simulink model "four_bots_CNN_DSM_compare"  (R2021a)
settings: Solver=ode5  StartTime=0.0  StopTime=30.0  FixedStep=0.001  RelTol=1e-3
(part 1 of 2)
settings Model: Creator=a1752760  LastModifiedBy=a1752760
settings SolverCC: AlgebraicLoopSolver=TrustRegion
settings DataIOCC: ReturnWorkspaceOutputs=off
settings DebuggingCC: SFMachineParentedDataDiag=warning  ArithmeticOperatorsInVariantConditions=warning
settings SFSimCC: CustomCodeUndefinedFunction=UseInterfaceOnly

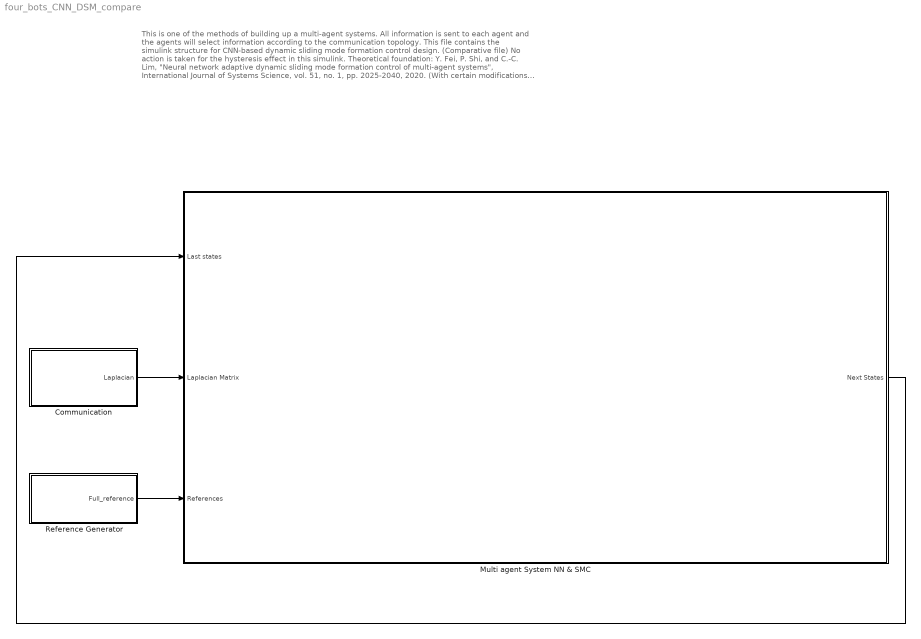
== system four_bots_CNN_DSM_compare ==
  note: This is one of the methods of building up a multi-agent systems. All information is sent to each agent and the agents will select information according to the communication topology.
      | This file contains the simulink structure for CNN-based dynamic sliding mode formation control design. (Comparative file)
      | No action is taken for the hysteresis effect in this simulink.
      | Theoretical foundation: Y. Fei, P. Shi, and C.-C. Lim, "Neural network adaptive dynamic sliding mode formation control of multi-agent systems", International Journal of Systems Science, vol. 51, no. 1, pp. 2025-2040, 2020. (With certain modifications in this simulink)
      | Note that some corrections have been made to the model (the system modelling and the formation reference part).
      | Copyright: Yang Fei @ The University of Adelaide 2021
  Communication : Subsystem
  Multi agent System NN & SMC : Subsystem
  Reference Generator : Subsystem
  wires:
  Communication/1(Laplacian) -> Multi agent System NN & SMC/2(Laplacian Matrix)
  Reference Generator/1(Full_reference) -> Multi agent System NN & SMC/3("References ")
  Multi agent System NN & SMC/1(Next States) -> Multi agent System NN & SMC/1(Last states)

== system four_bots_CNN_DSM_compare/Communication ==
  Add : Sum
  Communication Topology : Constant  Value=[2,-1,0,-1;-1,2,-1,0;0,-1,2,-1;-1,0,-1,2]  VectorParams1D=off
  Constant : Constant  Value=2  VectorParams1D=off
  Product : Product
  Reference Feeding : Constant  Value=[1,0,0,0;0,1,0,0;0,0,1,0;0,0,0,1]  VectorParams1D=off
  Laplacian : Outport  VectorParamsAs1DForOutWhenUnconnected=off
  wires:
  Constant/1 -> Product/2
  Reference Feeding/1 -> Product/1
  Communication Topology/1 -> Add/1
  Product/1 -> Add/2
  Add/1 -> Laplacian/1

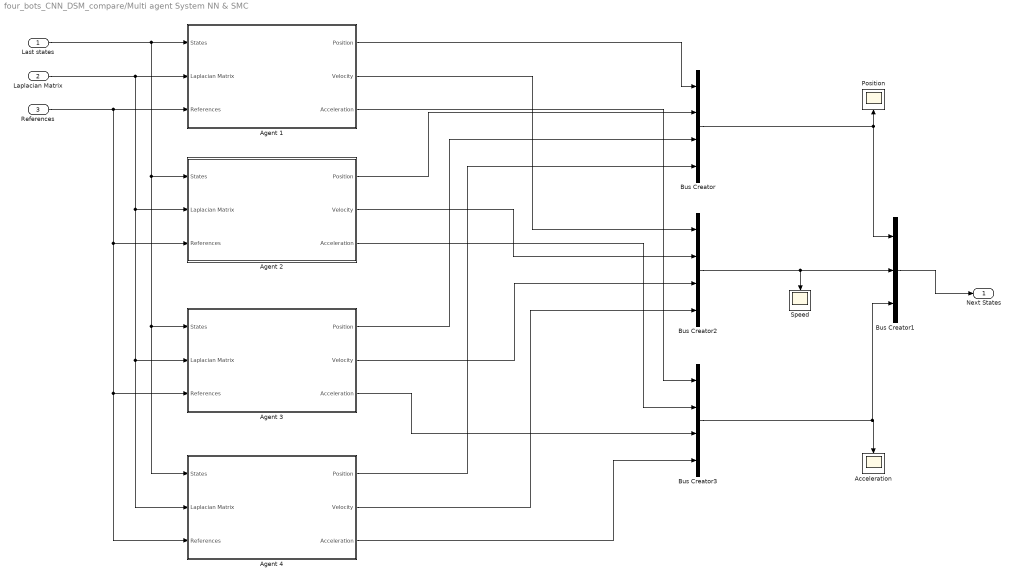
== system four_bots_CNN_DSM_compare/Multi agent System NN & SMC ==
  Last states : Inport
  Laplacian Matrix : Inport  Port=2
  "References " : Inport  Port=3
  Acceleration : Scope
  "Agent 1 " : Subsystem
  Agent 2 : Subsystem
  Agent 3 : Subsystem
  Agent 4 : Subsystem
  Bus Creator : BusCreator  Inputs=4
  Bus Creator1 : BusCreator  Inputs=3
  Bus Creator2 : BusCreator  Inputs=4
  Bus Creator3 : BusCreator  Inputs=4
  Position : Scope
  Speed : Scope
  Next States : Outport  VectorParamsAs1DForOutWhenUnconnected=off
  wires:
  Bus Creator1/1 -> Next States/1
  Last states/1 -> Agent 2/1(States), Agent 4/1(States), Agent 3/1(States), "Agent 1 "/1(States)
  Laplacian Matrix/1 -> Agent 2/2(Laplacian Matrix), Agent 4/2(Laplacian Matrix), Agent 3/2(Laplacian Matrix), "Agent 1 "/2(Laplacian Matrix)
  "References "/1 -> Agent 2/3("References "), Agent 4/3("References "), Agent 3/3("References "), "Agent 1 "/3("References ")
  "Agent 1 "/1(Position) -> Bus Creator/1
  Agent 2/1(Position) -> Bus Creator/2
  Agent 3/1(Position) -> Bus Creator/3
  Agent 4/1(Position) -> Bus Creator/4
  "Agent 1 "/2(Velocity) -> Bus Creator2/1
  Agent 2/2(Velocity) -> Bus Creator2/2
  Agent 3/2(Velocity) -> Bus Creator2/3
  Agent 4/2(Velocity) -> Bus Creator2/4
  "Agent 1 "/3(Acceleration) -> Bus Creator3/1
  Agent 2/3(Acceleration) -> Bus Creator3/2
  Agent 3/3(Acceleration) -> Bus Creator3/3
  Agent 4/3(Acceleration) -> Bus Creator3/4
  Bus Creator/1 -> Bus Creator1/1, Position/1
  Bus Creator2/1 -> Speed/1, Bus Creator1/2
  Bus Creator3/1 -> Bus Creator1/3, Acceleration/1

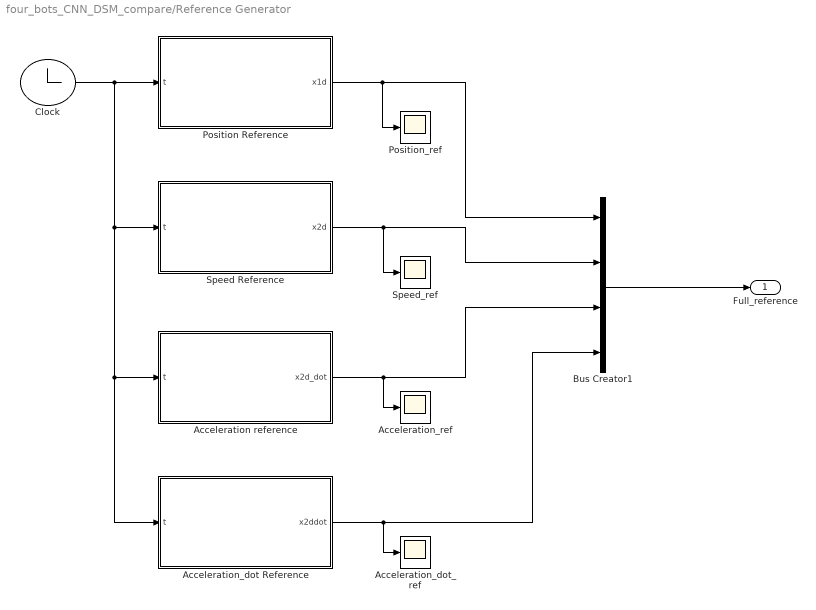
== system four_bots_CNN_DSM_compare/Reference Generator ==
  Acceleration reference : MATLAB Function  TreatAsAtomicUnit=on
  Acceleration_dot Reference : MATLAB Function  TreatAsAtomicUnit=on
  Acceleration_dot_ref : Scope
  Acceleration_ref : Scope
  Bus Creator1 : BusCreator  Inputs=4
  Clock : Clock
  Position Reference : MATLAB Function  TreatAsAtomicUnit=on
  Position_ref : Scope
  Speed Reference : MATLAB Function  TreatAsAtomicUnit=on
  Speed_ref : Scope
  Full_reference : Outport  VectorParamsAs1DForOutWhenUnconnected=off
  wires:
  Clock/1 -> Acceleration_dot Reference/1(t), Acceleration reference/1(t), Speed Reference/1(t), Position Reference/1(t)
  Position Reference/1(x1d) -> Position_ref/1, Bus Creator1/1
  Speed Reference/1(x2d) -> Speed_ref/1, Bus Creator1/2
  Acceleration reference/1(x2d_dot) -> Acceleration_ref/1, Bus Creator1/3
  Acceleration_dot Reference/1(x2ddot) -> Acceleration_dot_ref/1, Bus Creator1/4
  Bus Creator1/1 -> Full_reference/1

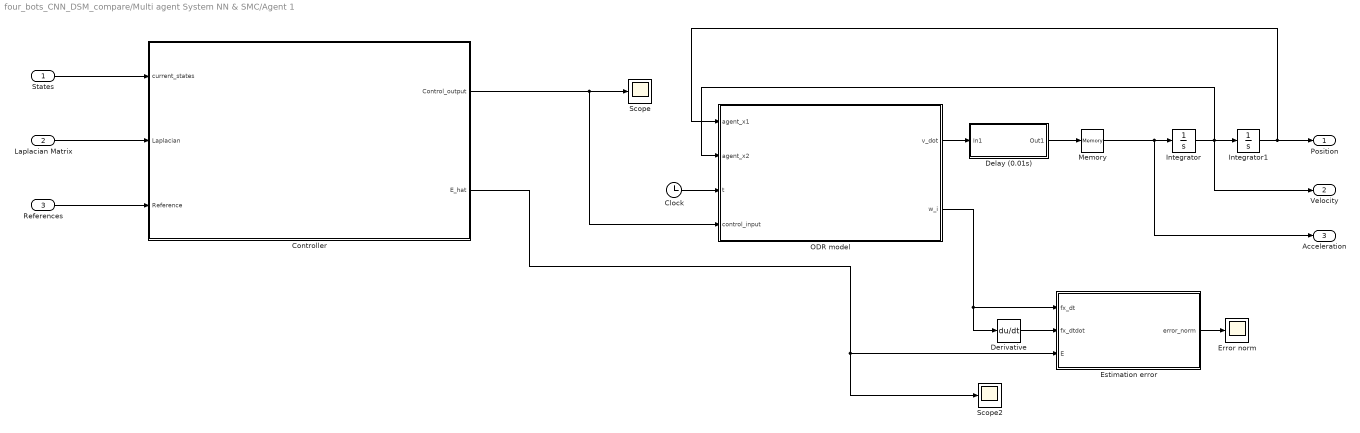
== system four_bots_CNN_DSM_compare/Multi agent System NN & SMC/Agent 1  ==
  States : Inport
  Laplacian Matrix : Inport  Port=2
  "References " : Inport  Port=3
  Clock : Clock
  "Controller " : Subsystem
  Delay (0.01s) : Subsystem
  Derivative : Derivative
  Error norm : Scope
  Estimation error : MATLAB Function  TreatAsAtomicUnit=on
  Integrator : Integrator  InitialCondition=[0;0;0]  ContinuousStateAttributes='speed'
  Integrator1 : Integrator  Tag=Position_x1  InitialCondition=[2;3;0]  ContinuousStateAttributes='position'
  Memory : Memory  InitialCondition=[0;0;0]  LinearizeMemory=on
  ODR model : MATLAB Function  TreatAsAtomicUnit=on
  Scope : Scope
  Scope2 : Scope
  Position : Outport  VectorParamsAs1DForOutWhenUnconnected=off
  Velocity : Outport  Port=2  VectorParamsAs1DForOutWhenUnconnected=off
  Acceleration : Outport  Port=3  VectorParamsAs1DForOutWhenUnconnected=off
  wires:
  ODR model/2(w_i) -> Estimation error/1(fx_dt), Derivative/1
  Integrator/1 -> ODR model/2(agent_x2), Velocity/1, Integrator1/1
  Integrator1/1 -> ODR model/1(agent_x1), Position/1
  ODR model/1(v_dot) -> Delay (0.01s)/1(In1)
  Delay (0.01s)/1(Out1) -> Memory/1
  States/1 -> "Controller "/1(current_states)
  Laplacian Matrix/1 -> "Controller "/2(Laplacian)
  "References "/1 -> "Controller "/3(Reference)
  "Controller "/1(Control_output) -> ODR model/4(control_input), Scope/1
  Clock/1 -> ODR model/3(t)
  Derivative/1 -> Estimation error/2(fx_dtdot)
  "Controller "/2(E_hat) -> Scope2/1, Estimation error/3(E)
  Estimation error/1(error_norm) -> Error norm/1
  Memory/1 -> Acceleration/1, Integrator/1

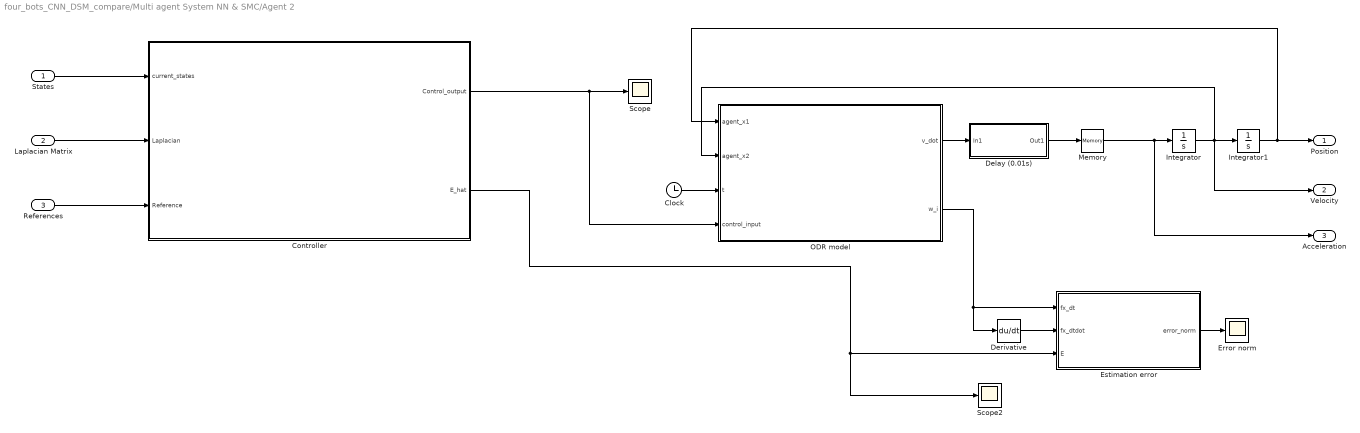
== system four_bots_CNN_DSM_compare/Multi agent System NN & SMC/Agent 2 ==
  States : Inport
  Laplacian Matrix : Inport  Port=2
  "References " : Inport  Port=3
  Clock : Clock
  "Controller " : Subsystem
  Delay (0.01s) : Subsystem
  Derivative : Derivative
  Error norm : Scope
  Estimation error : MATLAB Function  TreatAsAtomicUnit=on
  Integrator : Integrator  InitialCondition=[0;0;0]  ContinuousStateAttributes='speed'
  Integrator1 : Integrator  Tag=Position_x1  InitialCondition=[-0.5;2;pi/4]  ContinuousStateAttributes='position'
  Memory : Memory  InitialCondition=[0;0;0]  LinearizeMemory=on
  ODR model : MATLAB Function  TreatAsAtomicUnit=on
  Scope : Scope
  Scope2 : Scope
  Position : Outport  VectorParamsAs1DForOutWhenUnconnected=off
  Velocity : Outport  Port=2  VectorParamsAs1DForOutWhenUnconnected=off
  Acceleration : Outport  Port=3  VectorParamsAs1DForOutWhenUnconnected=off
  wires:
  ODR model/2(w_i) -> Estimation error/1(fx_dt), Derivative/1
  Integrator/1 -> ODR model/2(agent_x2), Velocity/1, Integrator1/1
  Integrator1/1 -> ODR model/1(agent_x1), Position/1
  ODR model/1(v_dot) -> Delay (0.01s)/1(In1)
  Delay (0.01s)/1(Out1) -> Memory/1
  States/1 -> "Controller "/1(current_states)
  Laplacian Matrix/1 -> "Controller "/2(Laplacian)
  "References "/1 -> "Controller "/3(Reference)
  "Controller "/1(Control_output) -> ODR model/4(control_input), Scope/1
  Clock/1 -> ODR model/3(t)
  Derivative/1 -> Estimation error/2(fx_dtdot)
  "Controller "/2(E_hat) -> Scope2/1, Estimation error/3(E)
  Estimation error/1(error_norm) -> Error norm/1
  Memory/1 -> Acceleration/1, Integrator/1

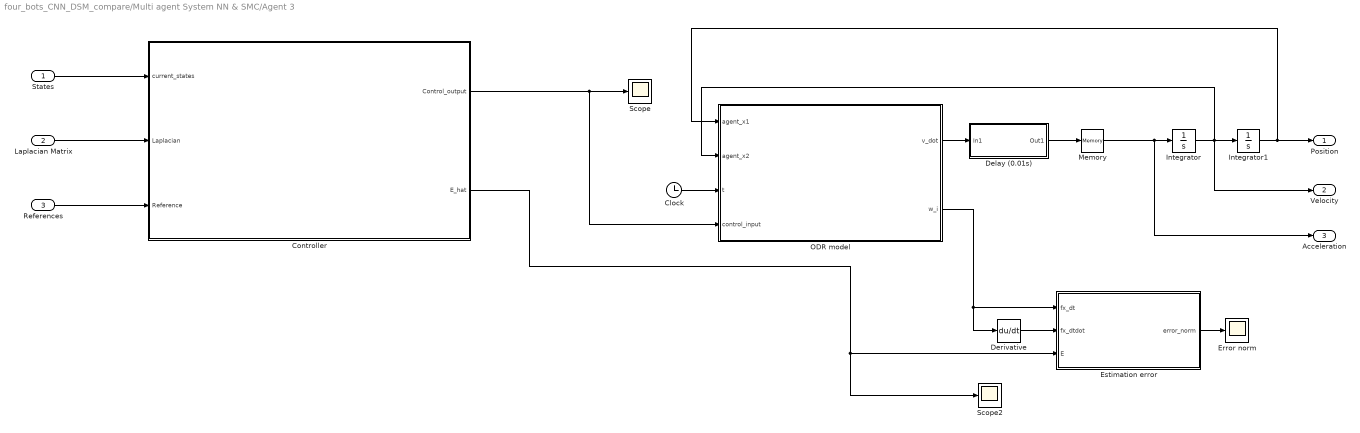
== system four_bots_CNN_DSM_compare/Multi agent System NN & SMC/Agent 3 ==
  States : Inport
  Laplacian Matrix : Inport  Port=2
  "References " : Inport  Port=3
  Clock : Clock
  "Controller " : Subsystem
  Delay (0.01s) : Subsystem
  Derivative : Derivative
  Error norm : Scope
  Estimation error : MATLAB Function  TreatAsAtomicUnit=on
  Integrator : Integrator  InitialCondition=[0;0;0]  ContinuousStateAttributes='speed'
  Integrator1 : Integrator  Tag=Position_x1  InitialCondition=[0.5;0;2*pi/3]  ContinuousStateAttributes='position'
  Memory : Memory  InitialCondition=[0;0;0]  LinearizeMemory=on
  ODR model : MATLAB Function  TreatAsAtomicUnit=on
  Scope : Scope
  Scope2 : Scope
  Position : Outport  VectorParamsAs1DForOutWhenUnconnected=off
  Velocity : Outport  Port=2  VectorParamsAs1DForOutWhenUnconnected=off
  Acceleration : Outport  Port=3  VectorParamsAs1DForOutWhenUnconnected=off
  wires:
  ODR model/2(w_i) -> Estimation error/1(fx_dt), Derivative/1
  Integrator/1 -> ODR model/2(agent_x2), Velocity/1, Integrator1/1
  Integrator1/1 -> ODR model/1(agent_x1), Position/1
  ODR model/1(v_dot) -> Delay (0.01s)/1(In1)
  Delay (0.01s)/1(Out1) -> Memory/1
  States/1 -> "Controller "/1(current_states)
  Laplacian Matrix/1 -> "Controller "/2(Laplacian)
  "References "/1 -> "Controller "/3(Reference)
  "Controller "/1(Control_output) -> ODR model/4(control_input), Scope/1
  Clock/1 -> ODR model/3(t)
  Derivative/1 -> Estimation error/2(fx_dtdot)
  "Controller "/2(E_hat) -> Scope2/1, Estimation error/3(E)
  Estimation error/1(error_norm) -> Error norm/1
  Memory/1 -> Acceleration/1, Integrator/1

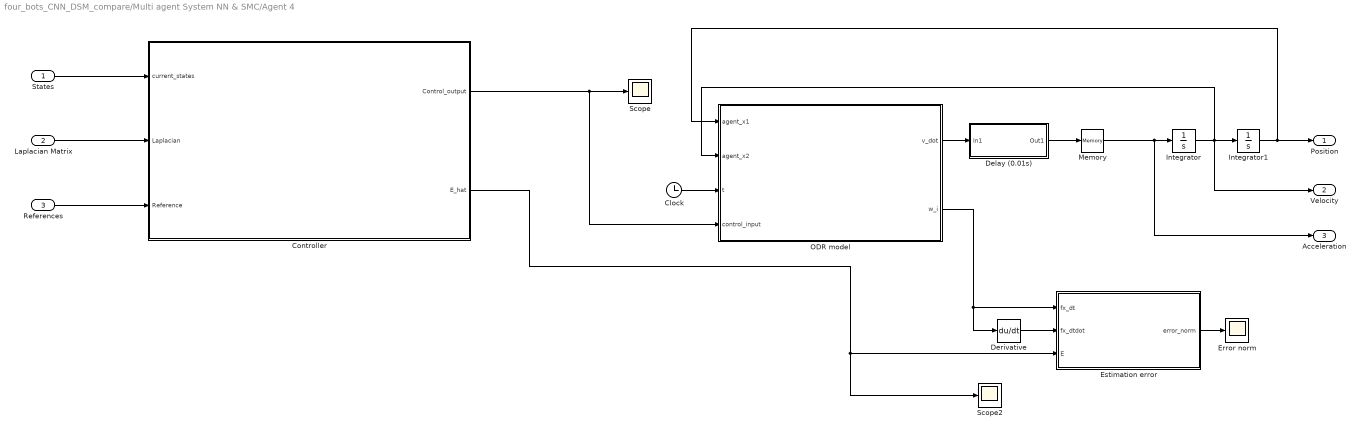
== system four_bots_CNN_DSM_compare/Multi agent System NN & SMC/Agent 4 ==
  States : Inport
  Laplacian Matrix : Inport  Port=2
  "References " : Inport  Port=3
  Clock : Clock
  "Controller " : Subsystem
  Delay (0.01s) : Subsystem
  Derivative : Derivative
  Error norm : Scope
  Estimation error : MATLAB Function  TreatAsAtomicUnit=on
  Integrator : Integrator  InitialCondition=[0;0;0]  ContinuousStateAttributes='speed'
  Integrator1 : Integrator  Tag=Position_x1  InitialCondition=[1.5;1;5*pi/4]  ContinuousStateAttributes='position'
  Memory : Memory  InitialCondition=[0;0;0]  LinearizeMemory=on
  ODR model : MATLAB Function  TreatAsAtomicUnit=on
  Scope : Scope
  Scope2 : Scope
  Position : Outport  VectorParamsAs1DForOutWhenUnconnected=off
  Velocity : Outport  Port=2  VectorParamsAs1DForOutWhenUnconnected=off
  Acceleration : Outport  Port=3  VectorParamsAs1DForOutWhenUnconnected=off
  wires:
  ODR model/2(w_i) -> Estimation error/1(fx_dt), Derivative/1
  Integrator/1 -> ODR model/2(agent_x2), Velocity/1, Integrator1/1
  Integrator1/1 -> ODR model/1(agent_x1), Position/1
  ODR model/1(v_dot) -> Delay (0.01s)/1(In1)
  Delay (0.01s)/1(Out1) -> Memory/1
  States/1 -> "Controller "/1(current_states)
  Laplacian Matrix/1 -> "Controller "/2(Laplacian)
  "References "/1 -> "Controller "/3(Reference)
  "Controller "/1(Control_output) -> ODR model/4(control_input), Scope/1
  Clock/1 -> ODR model/3(t)
  Derivative/1 -> Estimation error/2(fx_dtdot)
  "Controller "/2(E_hat) -> Scope2/1, Estimation error/3(E)
  Estimation error/1(error_norm) -> Error norm/1
  Memory/1 -> Acceleration/1, Integrator/1

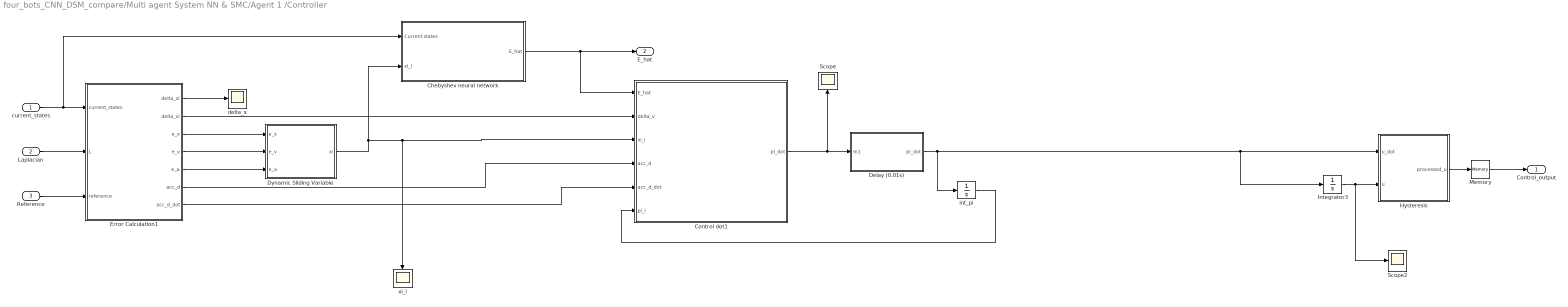
== system four_bots_CNN_DSM_compare/Multi agent System NN & SMC/Agent 1 /Controller  ==
  current_states : Inport
  Laplacian : Inport  Port=2
  Reference : Inport  Port=3
  Chebyshev neural network : Subsystem
  Control dot1 : MATLAB Function  TreatAsAtomicUnit=on
  Delay (0.01s) : Subsystem
  Dynamic Sliding Variable : MATLAB Function  TreatAsAtomicUnit=on
  Error Calculation1 : MATLAB Function  TreatAsAtomicUnit=on
  Hysteresis : Subsystem
  Integrator3 : Integrator  InitialCondition=[0;0;0]  UpperSaturationLimit=200  LowerSaturationLimit=-200  ContinuousStateAttributes='Control_output'
  Memory : Memory  InitialCondition=[0;0;0]  LinearizeMemory=on
  Scope : Scope
  Scope2 : Scope
  delta_x : Scope
  int_pi : Integrator  InitialCondition=[0;0;0]  UpperSaturationLimit=200  LowerSaturationLimit=-200  ContinuousStateAttributes='Control_output'
  xi_i : Scope
  Control_output : Outport
  E_hat : Outport  Port=2
  wires:
  Control dot1/1(pi_dot) -> Scope/1, Delay (0.01s)/1(In1)
  Hysteresis/1(processed_u) -> Memory/1
  Delay (0.01s)/1(pi_dot) -> Integrator3/1, Hysteresis/1(u_dot), int_pi/1
  Memory/1 -> Control_output/1
  Error Calculation1/4(e_v) -> Dynamic Sliding Variable/2(e_v)
  Laplacian/1 -> Error Calculation1/2(L)
  Error Calculation1/7(acc_d_dot) -> Control dot1/5(acc_d_dot)
  Error Calculation1/6(acc_d) -> Control dot1/4(acc_d)
  Reference/1 -> Error Calculation1/3(reference)
  Error Calculation1/5(e_a) -> Dynamic Sliding Variable/3(e_a)
  Error Calculation1/3(e_x) -> Dynamic Sliding Variable/1(e_x)
  Error Calculation1/2(delta_vi) -> Control dot1/2(delta_v)
  current_states/1 -> Chebyshev neural network/1(Current states), Error Calculation1/1(current_states)
  Error Calculation1/1(delta_xi) -> delta_x/1
  Dynamic Sliding Variable/1(xi) -> Control dot1/3(xi_i), xi_i/1, Chebyshev neural network/2(xi_i)
  Chebyshev neural network/1(E_hat) -> E_hat/1, Control dot1/1(E_hat)
  int_pi/1 -> Control dot1/6(pi_i)
  Integrator3/1 -> Scope2/1, Hysteresis/2(u)

== system four_bots_CNN_DSM_compare/Multi agent System NN & SMC/Agent 1 /Delay (0.01s) ==
  In1 : Inport
  Clock : Clock
  Constant : Constant  Value=[0;0;0]
  Scope3 : Scope
  Switch : Switch  Criteria=u2 > Threshold  Threshold=0.01
  Out1 : Outport  VectorParamsAs1DForOutWhenUnconnected=off
  wires:
  Constant/1 -> Switch/3
  In1/1 -> Switch/1
  Switch/1 -> Out1/1, Scope3/1
  Clock/1 -> Switch/2

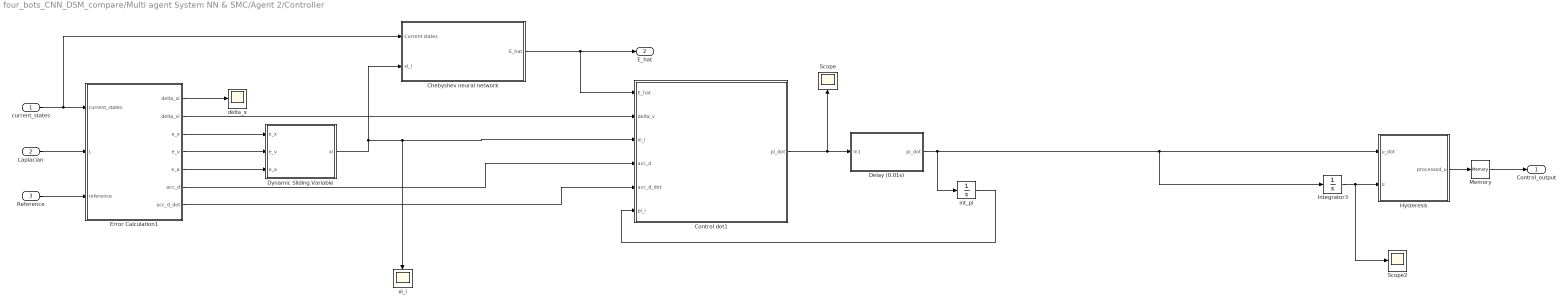
== system four_bots_CNN_DSM_compare/Multi agent System NN & SMC/Agent 2/Controller  ==
  current_states : Inport
  Laplacian : Inport  Port=2
  Reference : Inport  Port=3
  Chebyshev neural network : Subsystem
  Control dot1 : MATLAB Function  TreatAsAtomicUnit=on
  Delay (0.01s) : Subsystem
  Dynamic Sliding Variable : MATLAB Function  TreatAsAtomicUnit=on
  Error Calculation1 : MATLAB Function  TreatAsAtomicUnit=on
  Hysteresis : Subsystem
  Integrator3 : Integrator  InitialCondition=[0;0;0]  UpperSaturationLimit=200  LowerSaturationLimit=-200  ContinuousStateAttributes='Control_output'
  Memory : Memory  InitialCondition=[0;0;0]  LinearizeMemory=on
  Scope : Scope
  Scope2 : Scope
  delta_x : Scope
  int_pi : Integrator  InitialCondition=[0;0;0]  UpperSaturationLimit=200  LowerSaturationLimit=-200  ContinuousStateAttributes='Control_output'
  xi_i : Scope
  Control_output : Outport
  E_hat : Outport  Port=2
  wires:
  Control dot1/1(pi_dot) -> Scope/1, Delay (0.01s)/1(In1)
  Hysteresis/1(processed_u) -> Memory/1
  Delay (0.01s)/1(pi_dot) -> Integrator3/1, Hysteresis/1(u_dot), int_pi/1
  Memory/1 -> Control_output/1
  Error Calculation1/4(e_v) -> Dynamic Sliding Variable/2(e_v)
  Laplacian/1 -> Error Calculation1/2(L)
  Error Calculation1/7(acc_d_dot) -> Control dot1/5(acc_d_dot)
  Error Calculation1/6(acc_d) -> Control dot1/4(acc_d)
  Reference/1 -> Error Calculation1/3(reference)
  Error Calculation1/5(e_a) -> Dynamic Sliding Variable/3(e_a)
  Error Calculation1/3(e_x) -> Dynamic Sliding Variable/1(e_x)
  Error Calculation1/2(delta_vi) -> Control dot1/2(delta_v)
  current_states/1 -> Chebyshev neural network/1(Current states), Error Calculation1/1(current_states)
  Error Calculation1/1(delta_xi) -> delta_x/1
  Dynamic Sliding Variable/1(xi) -> Control dot1/3(xi_i), xi_i/1, Chebyshev neural network/2(xi_i)
  Chebyshev neural network/1(E_hat) -> E_hat/1, Control dot1/1(E_hat)
  int_pi/1 -> Control dot1/6(pi_i)
  Integrator3/1 -> Scope2/1, Hysteresis/2(u)

== system four_bots_CNN_DSM_compare/Multi agent System NN & SMC/Agent 2/Delay (0.01s) ==
  In1 : Inport
  Clock : Clock
  Constant : Constant  Value=[0;0;0]
  Scope3 : Scope
  Switch : Switch  Criteria=u2 > Threshold  Threshold=0.01
  Out1 : Outport  VectorParamsAs1DForOutWhenUnconnected=off
  wires:
  Constant/1 -> Switch/3
  In1/1 -> Switch/1
  Switch/1 -> Out1/1, Scope3/1
  Clock/1 -> Switch/2

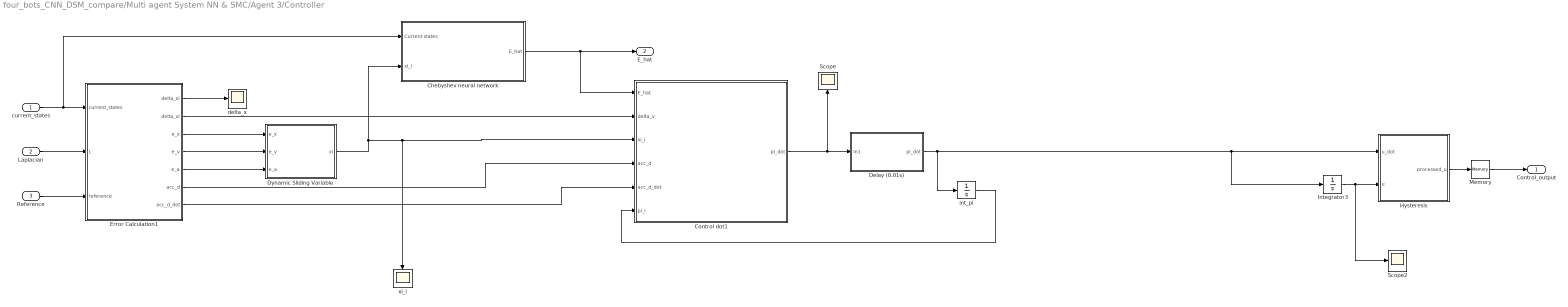
== system four_bots_CNN_DSM_compare/Multi agent System NN & SMC/Agent 3/Controller  ==
  current_states : Inport
  Laplacian : Inport  Port=2
  Reference : Inport  Port=3
  Chebyshev neural network : Subsystem
  Control dot1 : MATLAB Function  TreatAsAtomicUnit=on
  Delay (0.01s) : Subsystem
  Dynamic Sliding Variable : MATLAB Function  TreatAsAtomicUnit=on
  Error Calculation1 : MATLAB Function  TreatAsAtomicUnit=on
  Hysteresis : Subsystem
  Integrator3 : Integrator  InitialCondition=[0;0;0]  UpperSaturationLimit=200  LowerSaturationLimit=-200  ContinuousStateAttributes='Control_output'
  Memory : Memory  InitialCondition=[0;0;0]  LinearizeMemory=on
  Scope : Scope
  Scope2 : Scope
  delta_x : Scope
  int_pi : Integrator  InitialCondition=[0;0;0]  UpperSaturationLimit=200  LowerSaturationLimit=-200  ContinuousStateAttributes='Control_output'
  xi_i : Scope
  Control_output : Outport
  E_hat : Outport  Port=2
  wires:
  Control dot1/1(pi_dot) -> Scope/1, Delay (0.01s)/1(In1)
  Hysteresis/1(processed_u) -> Memory/1
  Delay (0.01s)/1(pi_dot) -> Integrator3/1, Hysteresis/1(u_dot), int_pi/1
  Memory/1 -> Control_output/1
  Error Calculation1/4(e_v) -> Dynamic Sliding Variable/2(e_v)
  Laplacian/1 -> Error Calculation1/2(L)
  Error Calculation1/7(acc_d_dot) -> Control dot1/5(acc_d_dot)
  Error Calculation1/6(acc_d) -> Control dot1/4(acc_d)
  Reference/1 -> Error Calculation1/3(reference)
  Error Calculation1/5(e_a) -> Dynamic Sliding Variable/3(e_a)
  Error Calculation1/3(e_x) -> Dynamic Sliding Variable/1(e_x)
  Error Calculation1/2(delta_vi) -> Control dot1/2(delta_v)
  current_states/1 -> Chebyshev neural network/1(Current states), Error Calculation1/1(current_states)
  Error Calculation1/1(delta_xi) -> delta_x/1
  Dynamic Sliding Variable/1(xi) -> Control dot1/3(xi_i), xi_i/1, Chebyshev neural network/2(xi_i)
  Chebyshev neural network/1(E_hat) -> E_hat/1, Control dot1/1(E_hat)
  int_pi/1 -> Control dot1/6(pi_i)
  Integrator3/1 -> Scope2/1, Hysteresis/2(u)

== system four_bots_CNN_DSM_compare/Multi agent System NN & SMC/Agent 3/Delay (0.01s) ==
  In1 : Inport
  Clock : Clock
  Constant : Constant  Value=[0;0;0]
  Scope3 : Scope
  Switch : Switch  Criteria=u2 > Threshold  Threshold=0.01
  Out1 : Outport  VectorParamsAs1DForOutWhenUnconnected=off
  wires:
  Constant/1 -> Switch/3
  In1/1 -> Switch/1
  Switch/1 -> Out1/1, Scope3/1
  Clock/1 -> Switch/2

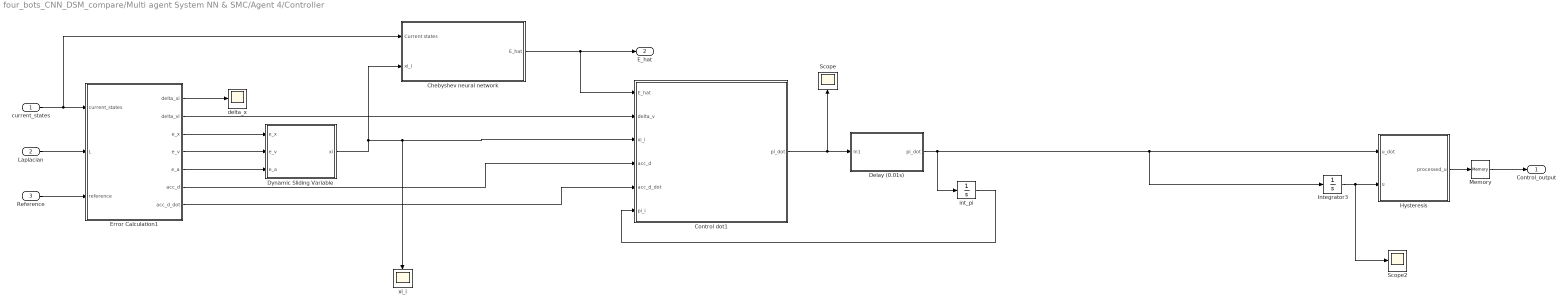
== system four_bots_CNN_DSM_compare/Multi agent System NN & SMC/Agent 4/Controller  ==
  current_states : Inport
  Laplacian : Inport  Port=2
  Reference : Inport  Port=3
  Chebyshev neural network : Subsystem
  Control dot1 : MATLAB Function  TreatAsAtomicUnit=on
  Delay (0.01s) : Subsystem
  Dynamic Sliding Variable : MATLAB Function  TreatAsAtomicUnit=on
  Error Calculation1 : MATLAB Function  TreatAsAtomicUnit=on
  Hysteresis : Subsystem
  Integrator3 : Integrator  InitialCondition=[0;0;0]  UpperSaturationLimit=200  LowerSaturationLimit=-200  ContinuousStateAttributes='Control_output'
  Memory : Memory  InitialCondition=[0;0;0]  LinearizeMemory=on
  Scope : Scope
  Scope2 : Scope
  delta_x : Scope
  int_pi : Integrator  InitialCondition=[0;0;0]  UpperSaturationLimit=200  LowerSaturationLimit=-200  ContinuousStateAttributes='Control_output'
  xi_i : Scope
  Control_output : Outport
  E_hat : Outport  Port=2
  wires:
  Control dot1/1(pi_dot) -> Scope/1, Delay (0.01s)/1(In1)
  Hysteresis/1(processed_u) -> Memory/1
  Delay (0.01s)/1(pi_dot) -> Hysteresis/1(u_dot), Integrator3/1, int_pi/1
  Memory/1 -> Control_output/1
  Error Calculation1/4(e_v) -> Dynamic Sliding Variable/2(e_v)
  Laplacian/1 -> Error Calculation1/2(L)
  Error Calculation1/7(acc_d_dot) -> Control dot1/5(acc_d_dot)
  Error Calculation1/6(acc_d) -> Control dot1/4(acc_d)
  Reference/1 -> Error Calculation1/3(reference)
  Error Calculation1/5(e_a) -> Dynamic Sliding Variable/3(e_a)
  Error Calculation1/3(e_x) -> Dynamic Sliding Variable/1(e_x)
  Error Calculation1/2(delta_vi) -> Control dot1/2(delta_v)
  current_states/1 -> Chebyshev neural network/1(Current states), Error Calculation1/1(current_states)
  Error Calculation1/1(delta_xi) -> delta_x/1
  Dynamic Sliding Variable/1(xi) -> Control dot1/3(xi_i), xi_i/1, Chebyshev neural network/2(xi_i)
  Chebyshev neural network/1(E_hat) -> E_hat/1, Control dot1/1(E_hat)
  int_pi/1 -> Control dot1/6(pi_i)
  Integrator3/1 -> Scope2/1, Hysteresis/2(u)

== system four_bots_CNN_DSM_compare/Multi agent System NN & SMC/Agent 4/Delay (0.01s) ==
  In1 : Inport
  Clock : Clock
  Constant : Constant  Value=[0;0;0]
  Scope3 : Scope
  Switch : Switch  Criteria=u2 > Threshold  Threshold=0.01
  Out1 : Outport  VectorParamsAs1DForOutWhenUnconnected=off
  wires:
  Constant/1 -> Switch/3
  In1/1 -> Switch/1
  Switch/1 -> Out1/1, Scope3/1
  Clock/1 -> Switch/2

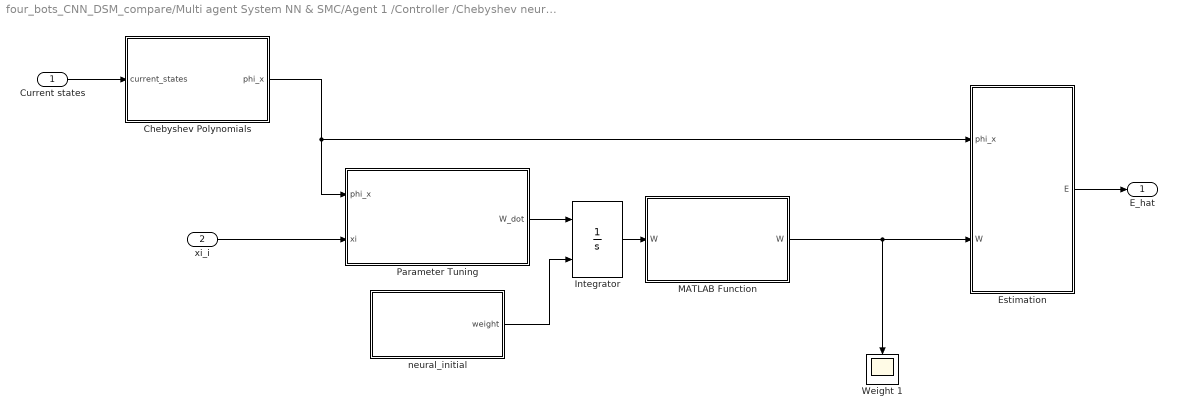
== system four_bots_CNN_DSM_compare/Multi agent System NN & SMC/Agent 1 /Controller /Chebyshev neural network ==
  Current states : Inport
  xi_i : Inport  Port=2
  Chebyshev Polynomials : MATLAB Function  TreatAsAtomicUnit=on
  Estimation : MATLAB Function  TreatAsAtomicUnit=on
  Integrator : Integrator  InitialConditionSource=external  InitialCondition=[0 0 0]'  UpperSaturationLimit=200  LowerSaturationLimit=-200  ContinuousStateAttributes='Neural_weights'
  MATLAB Function : MATLAB Function  TreatAsAtomicUnit=on
  Parameter Tuning : MATLAB Function  TreatAsAtomicUnit=on
  Weight 1 : Scope
  neural_initial : MATLAB Function  TreatAsAtomicUnit=on
  E_hat : Outport
  wires:
  MATLAB Function/1(W) -> Estimation/2(W), Weight 1/1
  Parameter Tuning/1(W_dot) -> Integrator/1
  neural_initial/1(weight) -> Integrator/2
  Integrator/1 -> MATLAB Function/1("W ")
  Chebyshev Polynomials/1(phi_x) -> Parameter Tuning/1(phi_x), Estimation/1(phi_x)
  Estimation/1(E) -> E_hat/1
  xi_i/1 -> Parameter Tuning/2(xi)
  Current states/1 -> Chebyshev Polynomials/1(current_states)

== system four_bots_CNN_DSM_compare/Multi agent System NN & SMC/Agent 1 /Controller /Delay (0.01s) ==
  In1 : Inport
  Clock : Clock
  Constant : Constant  Value=[0;0;0]
  Scope3 : Scope
  Switch : Switch  Criteria=u2 > Threshold  Threshold=0.01
  pi_dot : Outport  VectorParamsAs1DForOutWhenUnconnected=off
  wires:
  Constant/1 -> Switch/3
  In1/1 -> Switch/1
  Switch/1 -> pi_dot/1, Scope3/1
  Clock/1 -> Switch/2

== system four_bots_CNN_DSM_compare/Multi agent System NN & SMC/Agent 1 /Controller /Hysteresis ==
  u_dot : Inport
  u : Inport  Port=2
  Delay (0.01s) : Subsystem
  MATLAB Function1 : MATLAB Function  TreatAsAtomicUnit=on
  Scope1 : Scope
  zeta_int : Integrator  InitialCondition=[0;0;0]  ContinuousStateAttributes='speed'
  processed_u : Outport  VectorParamsAs1DForOutWhenUnconnected=off
  wires:
  zeta_int/1 -> MATLAB Function1/3(zeta)
  MATLAB Function1/2(zeta_dot) -> zeta_int/1, Scope1/1
  MATLAB Function1/1(actual_control) -> Delay (0.01s)/1(output)
  Delay (0.01s)/1(Out1) -> processed_u/1
  u/1 -> MATLAB Function1/1(u)
  u_dot/1 -> MATLAB Function1/2(u_dot)

== system four_bots_CNN_DSM_compare/Multi agent System NN & SMC/Agent 2/Controller /Chebyshev neural network ==
  Current states : Inport
  xi_i : Inport  Port=2
  Chebyshev Polynomials : MATLAB Function  TreatAsAtomicUnit=on
  Estimation : MATLAB Function  TreatAsAtomicUnit=on
  Integrator : Integrator  InitialConditionSource=external  InitialCondition=[0 0 0]'  UpperSaturationLimit=200  LowerSaturationLimit=-200  ContinuousStateAttributes='Neural_weights'
  MATLAB Function : MATLAB Function  TreatAsAtomicUnit=on
  Parameter Tuning : MATLAB Function  TreatAsAtomicUnit=on
  Weight 1 : Scope
  neural_initial : MATLAB Function  TreatAsAtomicUnit=on
  E_hat : Outport
  wires:
  MATLAB Function/1(W) -> Estimation/2(W), Weight 1/1
  Parameter Tuning/1(W_dot) -> Integrator/1
  neural_initial/1(weight) -> Integrator/2
  Integrator/1 -> MATLAB Function/1("W ")
  Chebyshev Polynomials/1(phi_x) -> Parameter Tuning/1(phi_x), Estimation/1(phi_x)
  Estimation/1(E) -> E_hat/1
  xi_i/1 -> Parameter Tuning/2(xi)
  Current states/1 -> Chebyshev Polynomials/1(current_states)

== system four_bots_CNN_DSM_compare/Multi agent System NN & SMC/Agent 2/Controller /Delay (0.01s) ==
  In1 : Inport
  Clock : Clock
  Constant : Constant  Value=[0;0;0]
  Scope3 : Scope
  Switch : Switch  Criteria=u2 > Threshold  Threshold=0.01
  pi_dot : Outport  VectorParamsAs1DForOutWhenUnconnected=off
  wires:
  Constant/1 -> Switch/3
  In1/1 -> Switch/1
  Switch/1 -> pi_dot/1, Scope3/1
  Clock/1 -> Switch/2

== system four_bots_CNN_DSM_compare/Multi agent System NN & SMC/Agent 2/Controller /Hysteresis ==
  u_dot : Inport
  u : Inport  Port=2
  Delay (0.01s) : Subsystem
  MATLAB Function1 : MATLAB Function  TreatAsAtomicUnit=on
  Scope1 : Scope
  zeta_int : Integrator  InitialCondition=[0;0;0]  ContinuousStateAttributes='speed'
  processed_u : Outport  VectorParamsAs1DForOutWhenUnconnected=off
  wires:
  zeta_int/1 -> MATLAB Function1/3(zeta)
  MATLAB Function1/2(zeta_dot) -> zeta_int/1, Scope1/1
  MATLAB Function1/1(actual_control) -> Delay (0.01s)/1(output)
  Delay (0.01s)/1(Out1) -> processed_u/1
  u/1 -> MATLAB Function1/1(u)
  u_dot/1 -> MATLAB Function1/2(u_dot)

== system four_bots_CNN_DSM_compare/Multi agent System NN & SMC/Agent 3/Controller /Chebyshev neural network ==
  Current states : Inport
  xi_i : Inport  Port=2
  Chebyshev Polynomials : MATLAB Function  TreatAsAtomicUnit=on
  Estimation : MATLAB Function  TreatAsAtomicUnit=on
  Integrator : Integrator  InitialConditionSource=external  InitialCondition=[0 0 0]'  UpperSaturationLimit=200  LowerSaturationLimit=-200  ContinuousStateAttributes='Neural_weights'
  MATLAB Function : MATLAB Function  TreatAsAtomicUnit=on
  Parameter Tuning : MATLAB Function  TreatAsAtomicUnit=on
  Weight 1 : Scope
  neural_initial : MATLAB Function  TreatAsAtomicUnit=on
  E_hat : Outport
  wires:
  MATLAB Function/1(W) -> Estimation/2(W), Weight 1/1
  Parameter Tuning/1(W_dot) -> Integrator/1
  neural_initial/1(weight) -> Integrator/2
  Integrator/1 -> MATLAB Function/1("W ")
  Chebyshev Polynomials/1(phi_x) -> Parameter Tuning/1(phi_x), Estimation/1(phi_x)
  Estimation/1(E) -> E_hat/1
  xi_i/1 -> Parameter Tuning/2(xi)
  Current states/1 -> Chebyshev Polynomials/1(current_states)

== system four_bots_CNN_DSM_compare/Multi agent System NN & SMC/Agent 3/Controller /Delay (0.01s) ==
  In1 : Inport
  Clock : Clock
  Constant : Constant  Value=[0;0;0]
  Scope3 : Scope
  Switch : Switch  Criteria=u2 > Threshold  Threshold=0.01
  pi_dot : Outport  VectorParamsAs1DForOutWhenUnconnected=off
  wires:
  Constant/1 -> Switch/3
  In1/1 -> Switch/1
  Switch/1 -> pi_dot/1, Scope3/1
  Clock/1 -> Switch/2

== system four_bots_CNN_DSM_compare/Multi agent System NN & SMC/Agent 3/Controller /Hysteresis ==
  u_dot : Inport
  u : Inport  Port=2
  Delay (0.01s) : Subsystem
  MATLAB Function1 : MATLAB Function  TreatAsAtomicUnit=on
  Scope1 : Scope
  zeta_int : Integrator  InitialCondition=[0;0;0]  ContinuousStateAttributes='speed'
  processed_u : Outport  VectorParamsAs1DForOutWhenUnconnected=off
  wires:
  zeta_int/1 -> MATLAB Function1/3(zeta)
  MATLAB Function1/2(zeta_dot) -> zeta_int/1, Scope1/1
  MATLAB Function1/1(actual_control) -> Delay (0.01s)/1(output)
  Delay (0.01s)/1(Out1) -> processed_u/1
  u/1 -> MATLAB Function1/1(u)
  u_dot/1 -> MATLAB Function1/2(u_dot)

== system four_bots_CNN_DSM_compare/Multi agent System NN & SMC/Agent 4/Controller /Chebyshev neural network ==
  Current states : Inport
  xi_i : Inport  Port=2
  Chebyshev Polynomials : MATLAB Function  TreatAsAtomicUnit=on
  Estimation : MATLAB Function  TreatAsAtomicUnit=on
  Integrator : Integrator  InitialConditionSource=external  InitialCondition=[0 0 0]'  UpperSaturationLimit=200  LowerSaturationLimit=-200  ContinuousStateAttributes='Neural_weights'
  MATLAB Function : MATLAB Function  TreatAsAtomicUnit=on
  Parameter Tuning : MATLAB Function  TreatAsAtomicUnit=on
  Weight 1 : Scope
  neural_initial : MATLAB Function  TreatAsAtomicUnit=on
  E_hat : Outport
  wires:
  MATLAB Function/1(W) -> Estimation/2(W), Weight 1/1
  Parameter Tuning/1(W_dot) -> Integrator/1
  neural_initial/1(weight) -> Integrator/2
  Integrator/1 -> MATLAB Function/1("W ")
  Chebyshev Polynomials/1(phi_x) -> Parameter Tuning/1(phi_x), Estimation/1(phi_x)
  Estimation/1(E) -> E_hat/1
  xi_i/1 -> Parameter Tuning/2(xi)
  Current states/1 -> Chebyshev Polynomials/1(current_states)

== system four_bots_CNN_DSM_compare/Multi agent System NN & SMC/Agent 4/Controller /Delay (0.01s) ==
  In1 : Inport
  Clock : Clock
  Constant : Constant  Value=[0;0;0]
  Scope3 : Scope
  Switch : Switch  Criteria=u2 > Threshold  Threshold=0.01
  pi_dot : Outport  VectorParamsAs1DForOutWhenUnconnected=off
  wires:
  Constant/1 -> Switch/3
  In1/1 -> Switch/1
  Switch/1 -> pi_dot/1, Scope3/1
  Clock/1 -> Switch/2

== system four_bots_CNN_DSM_compare/Multi agent System NN & SMC/Agent 4/Controller /Hysteresis ==
  u_dot : Inport
  u : Inport  Port=2
  Delay (0.01s) : Subsystem
  MATLAB Function1 : MATLAB Function  TreatAsAtomicUnit=on
  Scope1 : Scope
  zeta_int : Integrator  InitialCondition=[0;0;0]  ContinuousStateAttributes='speed'
  processed_u : Outport  VectorParamsAs1DForOutWhenUnconnected=off
  wires:
  zeta_int/1 -> MATLAB Function1/3(zeta)
  MATLAB Function1/2(zeta_dot) -> zeta_int/1, Scope1/1
  MATLAB Function1/1(actual_control) -> Delay (0.01s)/1(output)
  Delay (0.01s)/1(Out1) -> processed_u/1
  u/1 -> MATLAB Function1/1(u)
  u_dot/1 -> MATLAB Function1/2(u_dot)

== system four_bots_CNN_DSM_compare/Multi agent System NN & SMC/Agent 1 /Controller /Hysteresis/Delay (0.01s) ==
  output : Inport
  Clock : Clock
  Constant : Constant  Value=[0;0;0]
  Scope3 : Scope
  Switch : Switch  Criteria=u2 > Threshold  Threshold=0.01
  Out1 : Outport  VectorParamsAs1DForOutWhenUnconnected=off
  wires:
  Constant/1 -> Switch/3
  output/1 -> Switch/1
  Switch/1 -> Out1/1, Scope3/1
  Clock/1 -> Switch/2

== system four_bots_CNN_DSM_compare/Multi agent System NN & SMC/Agent 2/Controller /Hysteresis/Delay (0.01s) ==
  output : Inport
  Clock : Clock
  Constant : Constant  Value=[0;0;0]
  Scope3 : Scope
  Switch : Switch  Criteria=u2 > Threshold  Threshold=0.01
  Out1 : Outport  VectorParamsAs1DForOutWhenUnconnected=off
  wires:
  Constant/1 -> Switch/3
  output/1 -> Switch/1
  Switch/1 -> Out1/1, Scope3/1
  Clock/1 -> Switch/2

== system four_bots_CNN_DSM_compare/Multi agent System NN & SMC/Agent 3/Controller /Hysteresis/Delay (0.01s) ==
  output : Inport
  Clock : Clock
  Constant : Constant  Value=[0;0;0]
  Scope3 : Scope
  Switch : Switch  Criteria=u2 > Threshold  Threshold=0.01
  Out1 : Outport  VectorParamsAs1DForOutWhenUnconnected=off
  wires:
  Constant/1 -> Switch/3
  output/1 -> Switch/1
  Switch/1 -> Out1/1, Scope3/1
  Clock/1 -> Switch/2

== system four_bots_CNN_DSM_compare/Multi agent System NN & SMC/Agent 4/Controller /Hysteresis/Delay (0.01s) ==
  output : Inport
  Clock : Clock
  Constant : Constant  Value=[0;0;0]
  Scope3 : Scope
  Switch : Switch  Criteria=u2 > Threshold  Threshold=0.01
  Out1 : Outport  VectorParamsAs1DForOutWhenUnconnected=off
  wires:
  Constant/1 -> Switch/3
  output/1 -> Switch/1
  Switch/1 -> Out1/1, Scope3/1
  Clock/1 -> Switch/2

== matlab function four_bots_CNN_DSM_compare/Multi agent System NN & SMC/Agent 1 /Controller /Chebyshev neural network/Parameter Tuning ==
  data: phi_x input; xi input; W_dot output
function W_dot = parameter_tuning(phi_x, xi)

%% parameters that may alter
eta_1=0.1;

%% codes
W_dot = eta_1*phi_x*xi';

end

== matlab function four_bots_CNN_DSM_compare/Multi agent System NN & SMC/Agent 2/Controller /Control dot1 ==
  data: E_hat input; delta_v input; xi_i input; acc_d input; pi_dot output; acc_d_dot input; pi_i input
function pi_dot = control_dot(E_hat, delta_v, xi_i, acc_d, acc_d_dot , pi_i)

%% Basic parameters
dimension = 3;

%% Controller parameters
lambda = 2.5;
k = 2.5;
c = 10;

%% codes
pi_dot= -E_hat + acc_d_dot - (k + lambda) * (pi_i - acc_d) - k * lambda * delta_v - c * xi_i;

end

== matlab function four_bots_CNN_DSM_compare/Multi agent System NN & SMC/Agent 1 /Controller /Chebyshev neural network/neural_initial ==
  data: weight output
function weight = neural_initialize()

% cheby_order   : order of chebyshev polynomials
% dimension     : dimension of the system

cheby_order=3;
dimension=3;

weight = zeros(1+2*cheby_order*dimension, dimension);

end

== matlab function four_bots_CNN_DSM_compare/Multi agent System NN & SMC/Agent 2/Controller /Dynamic Sliding Variable ==
  data: e_x input; xi output; e_v input; e_a input
function xi = sliding_variable(e_x, e_v, e_a)

%% parameters that may alter
k=2.5;
lambda=2.5;

%% codes
xi = e_a + (k + lambda)* e_v + lambda * k * e_x;

end

== matlab function four_bots_CNN_DSM_compare/Multi agent System NN & SMC/Agent 2/Controller /Error Calculation1 ==
  data: current_states input; L input; delta_xi output; delta_vi output; reference input; e_x output; e_v output; e_a output; acc_d output; acc_d_dot output
function  [delta_xi, delta_vi, e_x, e_v, e_a, acc_d, acc_d_dot] = error_calculation(current_states, L, reference)

%% parameters that may change for alternative use
dimension = 3;
serial_num = 2;

num_agent = size(L,1);
%% current states
% Current states
pos = current_states(dimension*num_agent*0+1 : dimension*num_agent*1);
vel = current_states(dimension*num_agent*1+1 : dimension*num_agent*2);
acc = current_states(dimension*num_agent*2+1 : dimension*num_agent*3);

% Current reference
r_pos = reference(dimension*num_agent*0+1 : dimension*num_agent*1);
r_vel = reference(dimension*num_agent*1+1 : dimension*num_agent*2);
r_acc = reference(dimension*num_agent*2+1 : dimension*num_agent*3);
r_acc_dot = reference(dimension*num_agent*3+1 : dimension*num_agent*4);

%% Individual reference
acc_d = r_acc(dimension*(serial_num-1)+1 : dimension*serial_num);
acc_d_dot = r_acc_dot(dimension*(serial_num-1)+1 : dimension*serial_num);

%% Individual error
delta_x = pos - r_pos;
delta_v = vel - r_vel;

delta_xi = delta_x(dimension*(serial_num-1)+1 : dimension*serial_num);
delta_vi = delta_v(dimension*(serial_num-1)+1 : dimension*serial_num);

%% Local error
e_x = kron(L(serial_num, : ), eye(dimension) ) * (pos - r_pos);
e_v = kron(L(serial_num, : ), eye(dimension) ) * (vel - r_vel);
e_a = kron(L(serial_num, : ), eye(dimension) ) * (acc - r_acc);


end

== matlab function four_bots_CNN_DSM_compare/Multi agent System NN & SMC/Agent 2/Controller /Hysteresis/MATLAB Function1 ==
  data: u input; actual_control output; u_dot input; zeta input; zeta_dot output
function [actual_control, zeta_dot] = B_W_hysteresis(u, u_dot, zeta)

%% Hysteresis parameters
mu=1.5;
mu_bar=3;
chi_bar=1;
chi=0.5;
n=2;

actual_control=mu*u+mu_bar*zeta;

f=ones(3,1)-chi_bar*sign(u_dot).*abs(zeta).^(n-1).*zeta-chi*abs(zeta).^n;

zeta_dot=u_dot.*f;


end

== matlab function four_bots_CNN_DSM_compare/Multi agent System NN & SMC/Agent 2/Estimation error ==
  data: fx_dt input; error_norm output; fx_dtdot input; E input
function error_norm = estimation_error(fx_dt, fx_dtdot, E)

c=2.5;
lambda=2.5;

esti_error = fx_dtdot + (c + lambda) * fx_dt - E; 

error_norm = norm(esti_error); 

end

== matlab function four_bots_CNN_DSM_compare/Multi agent System NN & SMC/Agent 1 /Controller /Chebyshev neural network/Chebyshev Polynomials ==
  data: current_states input; phi_x output
function phi_x = Chebyshev_polynomials(current_states)

%% parameters that may alter
dimension=3;
cheby_order=3;

%% current states
x1=current_states(dimension*0+1:dimension*1);
x2=current_states(dimension*1+1:dimension*2);

%% initialization
phi_x=ones(1+2*dimension*cheby_order,1);

%% recursion procedure
now_x=[x1;x2];
for order = 1 : cheby_order
   if order == 1
      phi_x(2*dimension*(order-1)+2:2*dimension*order+1)=now_x;
   elseif order == 2
      phi_x(2*dimension*(order-1)+2:2*dimension*order+1)=2*now_x.*phi_x(2*dimension*(order-2)+2:2*dimension*(order-1)+1)-1;
   else
      phi_x(2*dimension*(order-1)+2:2*dimension*order+1)=2*now_x.*phi_x(2*dimension*(order-2)+2:2*dimension*(order-1)+1)-phi_x(2*dimension*(order-3)+2:2*dimension*(order-2)+1);
   end
end

end

== matlab function four_bots_CNN_DSM_compare/Multi agent System NN & SMC/Agent 2/ODR model ==
  data: agent_x1 input; v_dot output; agent_x2 input; t input; control_input input; w_i output
function [v_dot, w_i] = physical_model( agent_x1 , agent_x2, t, control_input )

Mass=[4.5,5.2,4.8,5.5];
Radius=[0.20,0.24,0.22,0.26];
Inertia=[2.2,2.4,2.3,2.5]/10;
Beta=[11.4,11.6,11.8,12.0];

%% assign the parameter according to serial number
serial_num = 2; 
m=Mass(serial_num);
R=Radius(serial_num);
inertia=Inertia(serial_num);
beta=Beta(serial_num);

%% current states of the robot
x=agent_x1(1);
y=agent_x1(2);
theta=agent_x1(3);

%% the real model of robot
M=diag([1/m,1/m,1/inertia]);
T=[-sin(theta), -sin(pi/3-theta), sin(pi/3+theta);
    cos(theta), -cos(pi/3-theta), -cos(pi/3+theta);
    R,          R,                  R];

T_R = [-sin(theta), -sin(pi/3-theta), sin(pi/3+theta);
        cos(theta), -cos(pi/3-theta), -cos(pi/3+theta);
        1/R,          1/R,                  1/R];

real_fx = - beta * T * T_R^(-1) * M * agent_x2;
% real_fx = zeros(3,1);
bar_w_i = [0.3 * x * sin(t+pi/3*serial_num)+2; 0.2 * y * cos(2*t+pi/3*serial_num)+1.5; 0.1 * theta * sin(0.8*t+pi/3*serial_num)+1];

%% saturation is added here for convinience
% Vmax=6; % the maximum voltage of the motor
% 
% u1up=Vmax/(alpha*m)*(abs(sin(theta))+abs(sin(pi/3-theta))+abs(sin(pi/3+theta)));
% u1do=-Vmax/(alpha*m)*(abs(sin(theta))+abs(sin(pi/3-theta))+abs(sin(pi/3+theta)));
% u2up=Vmax/(alpha*m)*(abs(cos(theta))+abs(cos(pi/3-theta))+abs(cos(pi/3+theta)));
% u2do=-Vmax/(alpha*m)*(abs(cos(theta))+abs(cos(pi/3-theta))+abs(cos(pi/3+theta)));
% u3up=R/(alpha*inertia)*3*Vmax;
% u3do=-R/(alpha*inertia)*3*Vmax;
% 
% control_input(1) = max( min(control_input(1),u1up), u1do );
% control_input(2) = max( min(control_input(2),u2up), u2do );
% control_input(3) = max( min(control_input(3),u3up), u3do );


w_i = real_fx + bar_w_i; 

v_dot = control_input + w_i;


end

== matlab function four_bots_CNN_DSM_compare/Multi agent System NN & SMC/Agent 1 /Estimation error ==
  data: fx_dt input; error_norm output; fx_dtdot input; E input
function error_norm = estimation_error(fx_dt, fx_dtdot, E)

c=2.5;
lambda=2.5;

esti_error = fx_dtdot + (c + lambda) * fx_dt - E; 

error_norm = norm(esti_error); 

end

== matlab function four_bots_CNN_DSM_compare/Multi agent System NN & SMC/Agent 3/Controller /Chebyshev neural network/Chebyshev Polynomials ==
  data: current_states input; phi_x output
function phi_x = Chebyshev_polynomials(current_states)

%% parameters that may alter
dimension=3;
cheby_order=3;

%% current states
x1=current_states(dimension*0+1:dimension*1);
x2=current_states(dimension*1+1:dimension*2);

%% initialization
phi_x=ones(1+2*dimension*cheby_order,1);

%% recursion procedure
now_x=[x1;x2];
for order = 1 : cheby_order
   if order == 1
      phi_x(2*dimension*(order-1)+2:2*dimension*order+1)=now_x;
   elseif order == 2
      phi_x(2*dimension*(order-1)+2:2*dimension*order+1)=2*now_x.*phi_x(2*dimension*(order-2)+2:2*dimension*(order-1)+1)-1;
   else
      phi_x(2*dimension*(order-1)+2:2*dimension*order+1)=2*now_x.*phi_x(2*dimension*(order-2)+2:2*dimension*(order-1)+1)-phi_x(2*dimension*(order-3)+2:2*dimension*(order-2)+1);
   end
end

end

== matlab function four_bots_CNN_DSM_compare/Multi agent System NN & SMC/Agent 3/Controller /Chebyshev neural network/Estimation ==
  data: phi_x input; W input; E output
function E = estimation(phi_x, W)
%% estimation
E=W'*phi_x;

end

== matlab function four_bots_CNN_DSM_compare/Multi agent System NN & SMC/Agent 3/Controller /Chebyshev neural network/MATLAB Function ==
  data: W input; W output
function W = smooth_projection(W)

%% smooth projection
Wmax=0.3;
Wmin=-0.3;
epsi=0.01;

for i=1:size(W,1)
   for j=1:size(W,2)
      if W(i,j)>Wmax
          W(i,j)=Wmax + epsi * (1-exp(-(W(i,j)-Wmax)/epsi));
      elseif W(i,j)<Wmin
          W(i,j)=Wmin - epsi * (1-exp((W(i,j)-Wmin)/epsi));
      else
          W(i,j)=W(i,j);
      end
   end
end

end

== matlab function four_bots_CNN_DSM_compare/Multi agent System NN & SMC/Agent 3/Controller /Chebyshev neural network/Parameter Tuning ==
  data: phi_x input; xi input; W_dot output
function W_dot = parameter_tuning(phi_x, xi)

%% parameters that may alter
eta_1=0.1;

%% codes
W_dot = eta_1*phi_x*xi';

end

== matlab function four_bots_CNN_DSM_compare/Multi agent System NN & SMC/Agent 3/Controller /Chebyshev neural network/neural_initial ==
  data: weight output
function weight = neural_initialize()

% cheby_order   : order of chebyshev polynomials
% dimension     : dimension of the system

cheby_order=3;
dimension=3;

weight = zeros(1+2*cheby_order*dimension, dimension);

end

== matlab function four_bots_CNN_DSM_compare/Multi agent System NN & SMC/Agent 3/Controller /Control dot1 ==
  data: E_hat input; delta_v input; xi_i input; acc_d input; pi_dot output; acc_d_dot input; pi_i input
function pi_dot = control_dot(E_hat, delta_v, xi_i, acc_d, acc_d_dot , pi_i)

%% Basic parameters
dimension = 3;

%% Controller parameters
lambda = 2.5;
k = 2.5;
c = 10;

%% codes
pi_dot= -E_hat + acc_d_dot - (k + lambda) * (pi_i - acc_d) - k * lambda * delta_v - c * xi_i;

end

== matlab function four_bots_CNN_DSM_compare/Multi agent System NN & SMC/Agent 3/Controller /Dynamic Sliding Variable ==
  data: e_x input; xi output; e_v input; e_a input
function xi = sliding_variable(e_x, e_v, e_a)

%% parameters that may alter
k=2.5;
lambda=2.5;

%% codes
xi = e_a + (k + lambda)* e_v + lambda * k * e_x;

end

== matlab function four_bots_CNN_DSM_compare/Multi agent System NN & SMC/Agent 1 /ODR model ==
  data: agent_x1 input; v_dot output; agent_x2 input; t input; control_input input; w_i output
function [v_dot, w_i] = physical_model( agent_x1 , agent_x2, t, control_input )

Mass=[4.5,5.2,4.8,5.5];
Radius=[0.20,0.24,0.22,0.26];
Inertia=[2.2,2.4,2.3,2.5]/10;
Beta=[11.4,11.6,11.8,12.0];

%% assign the parameter according to serial number
serial_num = 1; 
m=Mass(serial_num);
R=Radius(serial_num);
inertia=Inertia(serial_num);
beta=Beta(serial_num);

%% current states of the robot
x=agent_x1(1);
y=agent_x1(2);
theta=agent_x1(3);

%% the real model of robot
M=diag([1/m,1/m,1/inertia]);
T=[-sin(theta), -sin(pi/3-theta), sin(pi/3+theta);
    cos(theta), -cos(pi/3-theta), -cos(pi/3+theta);
    R,          R,                  R];

T_R = [-sin(theta), -sin(pi/3-theta), sin(pi/3+theta);
        cos(theta), -cos(pi/3-theta), -cos(pi/3+theta);
        1/R,          1/R,                  1/R];

real_fx = - beta * T * T_R^(-1) * M * agent_x2;
% real_fx = zeros(3,1);
bar_w_i = [0.3 * x * sin(t+pi/3*serial_num)+2; 0.2 * y * cos(2*t+pi/3*serial_num)+1.5; 0.1 * theta * sin(0.8*t+pi/3*serial_num)+1];

%% saturation is added here for convinience
% Vmax=6; % the maximum voltage of the motor
% 
% u1up=Vmax/(alpha*m)*(abs(sin(theta))+abs(sin(pi/3-theta))+abs(sin(pi/3+theta)));
% u1do=-Vmax/(alpha*m)*(abs(sin(theta))+abs(sin(pi/3-theta))+abs(sin(pi/3+theta)));
% u2up=Vmax/(alpha*m)*(abs(cos(theta))+abs(cos(pi/3-theta))+abs(cos(pi/3+theta)));
% u2do=-Vmax/(alpha*m)*(abs(cos(theta))+abs(cos(pi/3-theta))+abs(cos(pi/3+theta)));
% u3up=R/(alpha*inertia)*3*Vmax;
% u3do=-R/(alpha*inertia)*3*Vmax;
% 
% control_input(1) = max( min(control_input(1),u1up), u1do );
% control_input(2) = max( min(control_input(2),u2up), u2do );
% control_input(3) = max( min(control_input(3),u3up), u3do );


w_i = real_fx + bar_w_i; 

v_dot = control_input + w_i;


end

== matlab function four_bots_CNN_DSM_compare/Multi agent System NN & SMC/Agent 3/Controller /Error Calculation1 ==
  data: current_states input; L input; delta_xi output; delta_vi output; reference input; e_x output; e_v output; e_a output; acc_d output; acc_d_dot output
function  [delta_xi, delta_vi, e_x, e_v, e_a, acc_d, acc_d_dot] = error_calculation(current_states, L, reference)

%% parameters that may change for alternative use
dimension = 3;
serial_num = 3;

num_agent = size(L,1);
%% current states
% Current states
pos = current_states(dimension*num_agent*0+1 : dimension*num_agent*1);
vel = current_states(dimension*num_agent*1+1 : dimension*num_agent*2);
acc = current_states(dimension*num_agent*2+1 : dimension*num_agent*3);

% Current reference
r_pos = reference(dimension*num_agent*0+1 : dimension*num_agent*1);
r_vel = reference(dimension*num_agent*1+1 : dimension*num_agent*2);
r_acc = reference(dimension*num_agent*2+1 : dimension*num_agent*3);
r_acc_dot = reference(dimension*num_agent*3+1 : dimension*num_agent*4);

%% Individual reference
acc_d = r_acc(dimension*(serial_num-1)+1 : dimension*serial_num);
acc_d_dot = r_acc_dot(dimension*(serial_num-1)+1 : dimension*serial_num);

%% Individual error
delta_x = pos - r_pos;
delta_v = vel - r_vel;

delta_xi = delta_x(dimension*(serial_num-1)+1 : dimension*serial_num);
delta_vi = delta_v(dimension*(serial_num-1)+1 : dimension*serial_num);

%% Local error
e_x = kron(L(serial_num, : ), eye(dimension) ) * (pos - r_pos);
e_v = kron(L(serial_num, : ), eye(dimension) ) * (vel - r_vel);
e_a = kron(L(serial_num, : ), eye(dimension) ) * (acc - r_acc);


end

== matlab function four_bots_CNN_DSM_compare/Multi agent System NN & SMC/Agent 3/Controller /Hysteresis/MATLAB Function1 ==
  data: u input; actual_control output; u_dot input; zeta input; zeta_dot output
function [actual_control, zeta_dot] = B_W_hysteresis(u, u_dot, zeta)

%% Hysteresis parameters
mu=1.5;
mu_bar=3;
chi_bar=1;
chi=0.5;
n=2;

actual_control=mu*u+mu_bar*zeta;

f=ones(3,1)-chi_bar*sign(u_dot).*abs(zeta).^(n-1).*zeta-chi*abs(zeta).^n;

zeta_dot=u_dot.*f;


end

== matlab function four_bots_CNN_DSM_compare/Multi agent System NN & SMC/Agent 3/Estimation error ==
  data: fx_dt input; error_norm output; fx_dtdot input; E input
function error_norm = estimation_error(fx_dt, fx_dtdot, E)

c=2.5;
lambda=2.5;

esti_error = fx_dtdot + (c + lambda) * fx_dt - E; 

error_norm = norm(esti_error); 

end

== matlab function four_bots_CNN_DSM_compare/Multi agent System NN & SMC/Agent 3/ODR model ==
  data: agent_x1 input; v_dot output; agent_x2 input; t input; control_input input; w_i output
function [v_dot, w_i] = physical_model( agent_x1 , agent_x2, t, control_input )

Mass=[4.5,5.2,4.8,5.5];
Radius=[0.20,0.24,0.22,0.26];
Inertia=[2.2,2.4,2.3,2.5]/10;
Beta=[11.4,11.6,11.8,12.0];

%% assign the parameter according to serial number
serial_num = 3; 
m=Mass(serial_num);
R=Radius(serial_num);
inertia=Inertia(serial_num);
beta=Beta(serial_num);

%% current states of the robot
x=agent_x1(1);
y=agent_x1(2);
theta=agent_x1(3);

%% the real model of robot
M=diag([1/m,1/m,1/inertia]);
T=[-sin(theta), -sin(pi/3-theta), sin(pi/3+theta);
    cos(theta), -cos(pi/3-theta), -cos(pi/3+theta);
    R,          R,                  R];

T_R = [-sin(theta), -sin(pi/3-theta), sin(pi/3+theta);
        cos(theta), -cos(pi/3-theta), -cos(pi/3+theta);
        1/R,          1/R,                  1/R];

real_fx = - beta * T * T_R^(-1) * M * agent_x2;
% real_fx = zeros(3,1);
bar_w_i = [0.3 * x * sin(t+pi/3*serial_num)+2; 0.2 * y * cos(2*t+pi/3*serial_num)+1.5; 0.1 * theta * sin(0.8*t+pi/3*serial_num)+1];

%% saturation is added here for convinience
% Vmax=6; % the maximum voltage of the motor
% 
% u1up=Vmax/(alpha*m)*(abs(sin(theta))+abs(sin(pi/3-theta))+abs(sin(pi/3+theta)));
% u1do=-Vmax/(alpha*m)*(abs(sin(theta))+abs(sin(pi/3-theta))+abs(sin(pi/3+theta)));
% u2up=Vmax/(alpha*m)*(abs(cos(theta))+abs(cos(pi/3-theta))+abs(cos(pi/3+theta)));
% u2do=-Vmax/(alpha*m)*(abs(cos(theta))+abs(cos(pi/3-theta))+abs(cos(pi/3+theta)));
% u3up=R/(alpha*inertia)*3*Vmax;
% u3do=-R/(alpha*inertia)*3*Vmax;
% 
% control_input(1) = max( min(control_input(1),u1up), u1do );
% control_input(2) = max( min(control_input(2),u2up), u2do );
% control_input(3) = max( min(control_input(3),u3up), u3do );


w_i = real_fx + bar_w_i; 

v_dot = control_input + w_i;


end

== matlab function four_bots_CNN_DSM_compare/Multi agent System NN & SMC/Agent 4/Controller /Chebyshev neural network/Chebyshev Polynomials ==
  data: current_states input; phi_x output
function phi_x = Chebyshev_polynomials(current_states)

%% parameters that may alter
dimension=3;
cheby_order=3;

%% current states
x1=current_states(dimension*0+1:dimension*1);
x2=current_states(dimension*1+1:dimension*2);

%% initialization
phi_x=ones(1+2*dimension*cheby_order,1);

%% recursion procedure
now_x=[x1;x2];
for order = 1 : cheby_order
   if order == 1
      phi_x(2*dimension*(order-1)+2:2*dimension*order+1)=now_x;
   elseif order == 2
      phi_x(2*dimension*(order-1)+2:2*dimension*order+1)=2*now_x.*phi_x(2*dimension*(order-2)+2:2*dimension*(order-1)+1)-1;
   else
      phi_x(2*dimension*(order-1)+2:2*dimension*order+1)=2*now_x.*phi_x(2*dimension*(order-2)+2:2*dimension*(order-1)+1)-phi_x(2*dimension*(order-3)+2:2*dimension*(order-2)+1);
   end
end

end

== matlab function four_bots_CNN_DSM_compare/Multi agent System NN & SMC/Agent 4/Controller /Chebyshev neural network/Estimation ==
  data: phi_x input; W input; E output
function E = estimation(phi_x, W)
%% estimation
E=W'*phi_x;

end

== matlab function four_bots_CNN_DSM_compare/Multi agent System NN & SMC/Agent 4/Controller /Chebyshev neural network/MATLAB Function ==
  data: W input; W output
function W = smooth_projection(W)

%% smooth projection
Wmax=0.3;
Wmin=-0.3;
epsi=0.01;

for i=1:size(W,1)
   for j=1:size(W,2)
      if W(i,j)>Wmax
          W(i,j)=Wmax + epsi * (1-exp(-(W(i,j)-Wmax)/epsi));
      elseif W(i,j)<Wmin
          W(i,j)=Wmin - epsi * (1-exp((W(i,j)-Wmin)/epsi));
      else
          W(i,j)=W(i,j);
      end
   end
end

end
